simulink model "init_tank"  (R2018b)
settings: Solver=VariableStepAuto  StartTime=0.0  StopTime=100  FixedStep=0.0001  RelTol=1e-3
libraries: simulink x1
settings Model: Creator=Duc  LastModifiedBy=Duc

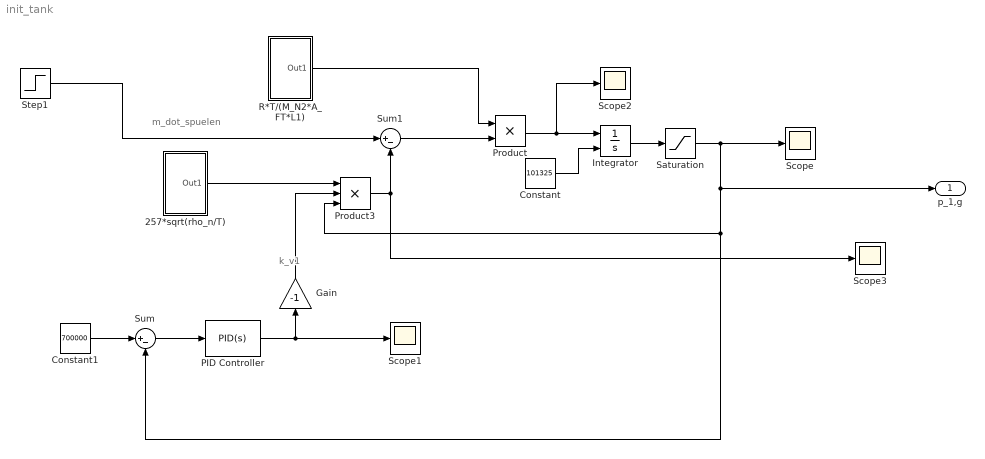
== system init_tank ==
  note: m_dot_spuelen
  note: k_v1
  257*sqrt(rho_n/T) : Subsystem
  Constant : Constant  Value=101325
  Constant1 : Constant  Value=700000
  Gain : Gain  Gain=-1
  Integrator : Integrator  InitialConditionSource=external  LowerSaturationLimit=0
  PID Controller : simulink/Continuous/PID Controller  Controller=PID  Form=Parallel  TimeDomain=Continuous-time  SampleTime=-1  IntegratorMethod=Forward Euler  FilterMethod=Forward Euler  ControllerParametersSource=internal  P=0.65  I=0.05  D=0.005  UseFilter=on  N=100  TunerSelectOption=Transfer Function Based (PID Tuner App)  InitialConditionSource=internal  InitialConditionForIntegrator=0  InitialConditionForFilter=0  DifferentiatorICPrevScaledInput=0  ExternalReset=none  TrackingMode=off  Kt=1  LimitOutput=on  UpperSaturationLimit=0  LowerSaturationLimit=-200  LinearizeAsGain=on  AntiWindupMode=clamping  Kb=1  POutMin=[]  POutMax=[]  IOutMin=[]  IOutMax=[]  DOutMin=[]  DOutMax=[]  NOutMin=[]  NOutMax=[]  SumOutMin=[]  SumOutMax=[]  SaturationOutMin=[]  SaturationOutMax=[]  PParamMin=[]  PParamMax=[]  IParamMin=[]  IParamMax=[]  DParamMin=[]  DParamMax=[]  NParamMin=[]  NParamMax=[]  KbParamMin=[]  KbParamMax=[]  KtParamMin=[]  KtParamMax=[]  KbOutMin=[]  KbOutMax=[]  KtOutMin=[]  KtOutMax=[]  IntegratorOutMin=[]  IntegratorOutMax=[]  FilterOutMin=[]  FilterOutMax=[]  SumI1OutMin=[]  SumI1OutMax=[]  SumI2OutMin=[]  SumI2OutMax=[]  SumI3OutMin=[]  SumI3OutMax=[]  SumI4OutMin=[]  SumI4OutMax=[]  SumDOutMin=[]  SumDOutMax=[]  DifferentiatorOutMin=[]  DifferentiatorOutMax=[]  FilterDiffOutCoefMin=[]  FilterDiffOutCoefMax=[]  ReciprocalOutMin=[]  ReciprocalOutMax=[]  SumDenOutMin=[]  SumDenOutMax=[]  SumNumOutMin=[]  SumNumOutMax=[]  DivideOutMin=[]  DivideOutMax=[]  IntegratorContinuousStateAttributes=''  IntegratorStateMustResolveToSignalObject=off  IntegratorRTWStateStorageClass=Auto  FilterContinuousStateAttributes=''  FilterStateMustResolveToSignalObject=off  FilterRTWStateStorageClass=Auto  ParallelPVariant=InternalParameters  IdealPVariant=Disabled  IVariant=InternalParameters  DVariant=InternalParameters  IntegratorVariant=Continuous  SatVariant=Enabled  AWVariant=ContClampingParallel  PCopyVariant=Disabled  TRVariant=Disabled  FdbkBlocksVariant=Forward  IdealPFdbkVariant=Disabled  SatFdbkVariant=Disabled  DerivativeFilterVariant=ContFilter  NVariant=InternalParameters  NCopyVariant=Disabled  FilterICVariant=InternalICsFilter  IntegratorICVariant=InternalICs  ExternalResetVariant=Disabled  TRSumVariant=Passthrough  SumFdbkVariant=Disabled  SumVariant=Sum_PID
  Product : Product
  Product3 : Product  Inputs=3
  R*T/(M_N2*A_FT*L1) : Subsystem
  Saturation : Saturate  UpperLimit=inf  LowerLimit=101325
  Scope{,1..3} (4 alike) : Scope
  Step1 : Step  After=0.1  SampleTime=0
  Sum : Sum  Inputs=|+-
  Sum1 : Sum  Inputs=|+-
  p_1,g : Outport
  wires:
  R*T/(M_N2*A_FT*L1)/1(Out1) -> Product/1
  Product/1 -> Scope2/1, Integrator/1
  Sum/1 -> PID Controller/1
  Constant1/1 -> Sum/1
  257*sqrt(rho_n/T)/1(Out1) -> Product3/1
  Step1/1 -> Sum1/1
  Product3/1 -> Sum1/2, Scope3/1
  Sum1/1 -> Product/2
  Constant/1 -> Integrator/2
  PID Controller/1 -> Scope1/1, Gain/1
  Integrator/1 -> Saturation/1
  Saturation/1 -> Scope/1, Product3/3, Sum/2, p_1,g/1
  Gain/1 -> Product3/2

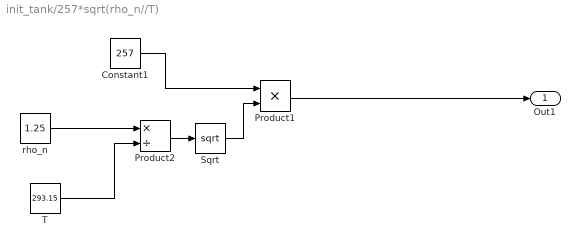
== system init_tank/257*sqrt(rho_n//T) ==
  Constant1 : Constant  Value=257
  Product1 : Product
  Product2 : Product  Inputs=*/
  Sqrt : Sqrt  SaturateOnIntegerOverflow=on
  T : Constant  Value=293.15
  rho_n : Constant  Value=1.25
  Out1 : Outport
  wires:
  Product2/1 -> Sqrt/1
  Product1/1 -> Out1/1
  Constant1/1 -> Product1/1
  T/1 -> Product2/2
  rho_n/1 -> Product2/1
  Sqrt/1 -> Product1/2

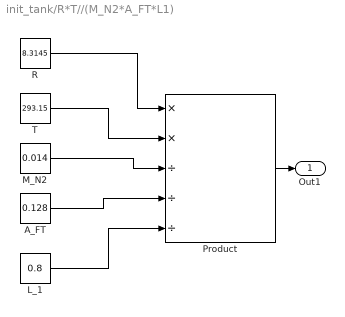
== system init_tank/R*T//(M_N2*A_FT*L1) ==
  A_FT : Constant  Value=0.128
  L_1 : Constant  Value=0.8
  M_N2 : Constant  Value=0.014
  Product : Product  Inputs=**///
  R : Constant  Value=8.3145
  T : Constant  Value=293.15
  Out1 : Outport
  wires:
  A_FT/1 -> Product/4
  M_N2/1 -> Product/3
  Product/1 -> Out1/1
  L_1/1 -> Product/5
  T/1 -> Product/2
  R/1 -> Product/1
